simulink model "w2_warplab_trigger_proc"  (Simulink 7.7)
settings: Solver=ode45  StartTime=0.0  StopTime=1000  RelTol=1e-3
InitFcn:
  | w2_warplab_trigger_proc_init
StartFcn:
  | w2_warplab_trigger_proc_init
undefined symbols (not defined in the file or in its folder): gcbh, xlBlockLoadCallback, xlGetNormalizedPeriod
libraries: xbsIndex_r4 x819, simulink x1
(part 5 of 6)

== system w2_warplab_trigger_proc/Registers/Output Configuration Slice9 ==
  32b : Inport
  b0 : xbsIndex_r4/Slice  nbits=1  boolean_output=off  mode=Lower Bit Location + Width  bit1=0  base1=MSB of Input  bit0=0  base0=LSB of Input  dbl_ovrd=off  block_type=slice
  b1 : xbsIndex_r4/Slice  nbits=1  boolean_output=off  mode=Lower Bit Location + Width  bit1=0  base1=MSB of Input  bit0=1  base0=LSB of Input  dbl_ovrd=off  block_type=slice
  b16 : xbsIndex_r4/Slice  nbits=1  boolean_output=off  mode=Lower Bit Location + Width  bit1=0  base1=MSB of Input  bit0=16  base0=LSB of Input  dbl_ovrd=off  block_type=slice
  b17 : xbsIndex_r4/Slice  nbits=1  boolean_output=off  mode=Lower Bit Location + Width  bit1=0  base1=MSB of Input  bit0=17  base0=LSB of Input  dbl_ovrd=off  block_type=slice
  b18 : xbsIndex_r4/Slice  nbits=1  boolean_output=off  mode=Lower Bit Location + Width  bit1=0  base1=MSB of Input  bit0=18  base0=LSB of Input  dbl_ovrd=off  block_type=slice
  b19 : xbsIndex_r4/Slice  nbits=1  boolean_output=off  mode=Lower Bit Location + Width  bit1=0  base1=MSB of Input  bit0=19  base0=LSB of Input  dbl_ovrd=off  block_type=slice
  b2 : xbsIndex_r4/Slice  nbits=1  boolean_output=off  mode=Lower Bit Location + Width  bit1=0  base1=MSB of Input  bit0=2  base0=LSB of Input  dbl_ovrd=off  block_type=slice
  b20 : xbsIndex_r4/Slice  nbits=1  boolean_output=off  mode=Lower Bit Location + Width  bit1=0  base1=MSB of Input  bit0=20  base0=LSB of Input  dbl_ovrd=off  block_type=slice
  b21 : xbsIndex_r4/Slice  nbits=1  boolean_output=off  mode=Lower Bit Location + Width  bit1=0  base1=MSB of Input  bit0=21  base0=LSB of Input  dbl_ovrd=off  block_type=slice
  b22 : xbsIndex_r4/Slice  nbits=1  boolean_output=off  mode=Lower Bit Location + Width  bit1=0  base1=MSB of Input  bit0=22  base0=LSB of Input  dbl_ovrd=off  block_type=slice
  b23 : xbsIndex_r4/Slice  nbits=1  boolean_output=off  mode=Lower Bit Location + Width  bit1=0  base1=MSB of Input  bit0=23  base0=LSB of Input  dbl_ovrd=off  block_type=slice
  b24 : xbsIndex_r4/Slice  nbits=1  boolean_output=off  mode=Lower Bit Location + Width  bit1=0  base1=MSB of Input  bit0=24  base0=LSB of Input  dbl_ovrd=off  block_type=slice
  b3 : xbsIndex_r4/Slice  nbits=1  boolean_output=off  mode=Lower Bit Location + Width  bit1=0  base1=MSB of Input  bit0=3  base0=LSB of Input  dbl_ovrd=off  block_type=slice
  b4 : xbsIndex_r4/Slice  nbits=1  boolean_output=off  mode=Lower Bit Location + Width  bit1=0  base1=MSB of Input  bit0=4  base0=LSB of Input  dbl_ovrd=off  block_type=slice
  b5 : xbsIndex_r4/Slice  nbits=1  boolean_output=off  mode=Lower Bit Location + Width  bit1=0  base1=MSB of Input  bit0=5  base0=LSB of Input  dbl_ovrd=off  block_type=slice
  b6 : xbsIndex_r4/Slice  nbits=1  boolean_output=off  mode=Lower Bit Location + Width  bit1=0  base1=MSB of Input  bit0=6  base0=LSB of Input  dbl_ovrd=off  block_type=slice
  b7 : xbsIndex_r4/Slice  nbits=1  boolean_output=off  mode=Lower Bit Location + Width  bit1=0  base1=MSB of Input  bit0=7  base0=LSB of Input  dbl_ovrd=off  block_type=slice
  b8 : xbsIndex_r4/Slice  nbits=1  boolean_output=off  mode=Lower Bit Location + Width  bit1=0  base1=MSB of Input  bit0=8  base0=LSB of Input  dbl_ovrd=off  block_type=slice
  bool{1..18} (18 alike) : xbsIndex_r4/Convert  gui_display_data_type=Boolean  arith_type=Boolean  n_bits=16  bin_pt=14  float_type=Single  exp_bits=8  fraction_bits=24  quantization=Truncate  overflow=Wrap  en=off  latency=0  dbl_ovrd=off  pipeline=off  block_type=convert
  AND 0 : Outport
  AND 1 : Outport  Port=2
  AND 2 : Outport  Port=3
  AND 3 : Outport  Port=4
  AND 4 : Outport  Port=5
  AND 5 : Outport  Port=6
  AND 6 : Outport  Port=7
  AND 7 : Outport  Port=8
  AND 8 : Outport  Port=9
  OR 0 : Outport  Port=10
  OR 1 : Outport  Port=11
  OR 2 : Outport  Port=12
  OR 3 : Outport  Port=13
  OR 4 : Outport  Port=14
  OR 5 : Outport  Port=15
  OR 6 : Outport  Port=16
  OR 7 : Outport  Port=17
  OR 8 : Outport  Port=18
  wires:
  32b/1 -> b0/1, b1/1, b2/1, b3/1, b4/1, b5/1, b6/1, b7/1, b16/1, b17/1, b18/1, b19/1, b20/1, b21/1, b22/1, b23/1, b24/1, b8/1
  b0/1 -> bool2/1
  b1/1 -> bool1/1
  b2/1 -> bool3/1
  b3/1 -> bool4/1
  b4/1 -> bool5/1
  b5/1 -> bool6/1
  b6/1 -> bool7/1
  b7/1 -> bool8/1
  b16/1 -> bool9/1
  b17/1 -> bool10/1
  b18/1 -> bool11/1
  b19/1 -> bool12/1
  b20/1 -> bool13/1
  b21/1 -> bool14/1
  b22/1 -> bool15/1
  b23/1 -> bool16/1
  bool2/1 -> AND 0/1
  bool1/1 -> AND 1/1
  bool3/1 -> AND 2/1
  bool4/1 -> AND 3/1
  bool5/1 -> AND 4/1
  bool6/1 -> AND 5/1
  bool7/1 -> AND 6/1
  bool8/1 -> AND 7/1
  bool9/1 -> OR 0/1
  bool10/1 -> OR 1/1
  bool11/1 -> OR 2/1
  bool12/1 -> OR 3/1
  bool13/1 -> OR 4/1
  bool14/1 -> OR 5/1
  bool15/1 -> OR 6/1
  bool16/1 -> OR 7/1
  b8/1 -> bool17/1
  bool17/1 -> AND 8/1
  b24/1 -> bool18/1
  bool18/1 -> OR 8/1

== system w2_warplab_trigger_proc/Trigger Output 0/S-R Latch ==
  S : Inport
  R : Inport  Port=2
  Constant1 : xbsIndex_r4/Constant  const=1  gui_display_data_type=Fixed-point  arith_type=Unsigned  n_bits=1  bin_pt=0  preci_type=Single  exp_width=8  frac_width=24  explicit_period=off  period=1  equ=P=C  opselect=C  inp2=PCIN>>17  opr=+  inp1=P  carry=CIN  dbl_ovrd=off  block_type=constant
      settings: block_version=VER_STRING_GOES_HERE
  Convert1 : xbsIndex_r4/Convert  gui_display_data_type=Boolean  arith_type=Boolean  n_bits=16  bin_pt=14  float_type=Single  exp_bits=8  fraction_bits=24  quantization=Truncate  overflow=Wrap  en=off  latency=0  dbl_ovrd=off  pipeline=off  block_type=convert
  Convert2 : xbsIndex_r4/Convert  gui_display_data_type=Boolean  arith_type=Boolean  n_bits=16  bin_pt=14  float_type=Single  exp_bits=8  fraction_bits=24  quantization=Truncate  overflow=Wrap  en=off  latency=0  dbl_ovrd=off  pipeline=off  block_type=convert
  Register2 : xbsIndex_r4/Register  init=0  rst=on  en=on  dbl_ovrd=off  block_type=register
      settings: xl_area=[1 1 0 0 0 0 0]  block_version=VER_STRING_GOES_HERE
  Q : Outport
  wires:
  S/1 -> Convert2/1
  Register2/1 -> Q/1
  R/1 -> Convert1/1
  Constant1/1 -> Register2/1
  Convert1/1 -> Register2/2
  Convert2/1 -> Register2/3

== system w2_warplab_trigger_proc/Trigger Output 1/S-R Latch ==
  S : Inport
  R : Inport  Port=2
  Constant1 : xbsIndex_r4/Constant  const=1  gui_display_data_type=Fixed-point  arith_type=Unsigned  n_bits=1  bin_pt=0  preci_type=Single  exp_width=8  frac_width=24  explicit_period=off  period=1  equ=P=C  opselect=C  inp2=PCIN>>17  opr=+  inp1=P  carry=CIN  dbl_ovrd=off  block_type=constant
      settings: block_version=VER_STRING_GOES_HERE
  Convert1 : xbsIndex_r4/Convert  gui_display_data_type=Boolean  arith_type=Boolean  n_bits=16  bin_pt=14  float_type=Single  exp_bits=8  fraction_bits=24  quantization=Truncate  overflow=Wrap  en=off  latency=0  dbl_ovrd=off  pipeline=off  block_type=convert
  Convert2 : xbsIndex_r4/Convert  gui_display_data_type=Boolean  arith_type=Boolean  n_bits=16  bin_pt=14  float_type=Single  exp_bits=8  fraction_bits=24  quantization=Truncate  overflow=Wrap  en=off  latency=0  dbl_ovrd=off  pipeline=off  block_type=convert
  Register2 : xbsIndex_r4/Register  init=0  rst=on  en=on  dbl_ovrd=off  block_type=register
      settings: xl_area=[1 1 0 0 0 0 0]  block_version=VER_STRING_GOES_HERE
  Q : Outport
  wires:
  S/1 -> Convert2/1
  Register2/1 -> Q/1
  R/1 -> Convert1/1
  Constant1/1 -> Register2/1
  Convert1/1 -> Register2/2
  Convert2/1 -> Register2/3

== system w2_warplab_trigger_proc/Trigger Output 2/S-R Latch ==
  S : Inport
  R : Inport  Port=2
  Constant1 : xbsIndex_r4/Constant  const=1  gui_display_data_type=Fixed-point  arith_type=Unsigned  n_bits=1  bin_pt=0  preci_type=Single  exp_width=8  frac_width=24  explicit_period=off  period=1  equ=P=C  opselect=C  inp2=PCIN>>17  opr=+  inp1=P  carry=CIN  dbl_ovrd=off  block_type=constant
      settings: block_version=VER_STRING_GOES_HERE
  Convert1 : xbsIndex_r4/Convert  gui_display_data_type=Boolean  arith_type=Boolean  n_bits=16  bin_pt=14  float_type=Single  exp_bits=8  fraction_bits=24  quantization=Truncate  overflow=Wrap  en=off  latency=0  dbl_ovrd=off  pipeline=off  block_type=convert
  Convert2 : xbsIndex_r4/Convert  gui_display_data_type=Boolean  arith_type=Boolean  n_bits=16  bin_pt=14  float_type=Single  exp_bits=8  fraction_bits=24  quantization=Truncate  overflow=Wrap  en=off  latency=0  dbl_ovrd=off  pipeline=off  block_type=convert
  Register2 : xbsIndex_r4/Register  init=0  rst=on  en=on  dbl_ovrd=off  block_type=register
      settings: xl_area=[1 1 0 0 0 0 0]  block_version=VER_STRING_GOES_HERE
  Q : Outport
  wires:
  S/1 -> Convert2/1
  Register2/1 -> Q/1
  R/1 -> Convert1/1
  Constant1/1 -> Register2/1
  Convert1/1 -> Register2/2
  Convert2/1 -> Register2/3

== system w2_warplab_trigger_proc/Trigger Output 3/S-R Latch ==
  S : Inport
  R : Inport  Port=2
  Constant1 : xbsIndex_r4/Constant  const=1  gui_display_data_type=Fixed-point  arith_type=Unsigned  n_bits=1  bin_pt=0  preci_type=Single  exp_width=8  frac_width=24  explicit_period=off  period=1  equ=P=C  opselect=C  inp2=PCIN>>17  opr=+  inp1=P  carry=CIN  dbl_ovrd=off  block_type=constant
      settings: block_version=VER_STRING_GOES_HERE
  Convert1 : xbsIndex_r4/Convert  gui_display_data_type=Boolean  arith_type=Boolean  n_bits=16  bin_pt=14  float_type=Single  exp_bits=8  fraction_bits=24  quantization=Truncate  overflow=Wrap  en=off  latency=0  dbl_ovrd=off  pipeline=off  block_type=convert
  Convert2 : xbsIndex_r4/Convert  gui_display_data_type=Boolean  arith_type=Boolean  n_bits=16  bin_pt=14  float_type=Single  exp_bits=8  fraction_bits=24  quantization=Truncate  overflow=Wrap  en=off  latency=0  dbl_ovrd=off  pipeline=off  block_type=convert
  Register2 : xbsIndex_r4/Register  init=0  rst=on  en=on  dbl_ovrd=off  block_type=register
      settings: xl_area=[1 1 0 0 0 0 0]  block_version=VER_STRING_GOES_HERE
  Q : Outport
  wires:
  S/1 -> Convert2/1
  Register2/1 -> Q/1
  R/1 -> Convert1/1
  Constant1/1 -> Register2/1
  Convert1/1 -> Register2/2
  Convert2/1 -> Register2/3

== system w2_warplab_trigger_proc/Trigger Output 4/S-R Latch ==
  S : Inport
  R : Inport  Port=2
  Constant1 : xbsIndex_r4/Constant  const=1  gui_display_data_type=Fixed-point  arith_type=Unsigned  n_bits=1  bin_pt=0  preci_type=Single  exp_width=8  frac_width=24  explicit_period=off  period=1  equ=P=C  opselect=C  inp2=PCIN>>17  opr=+  inp1=P  carry=CIN  dbl_ovrd=off  block_type=constant
      settings: block_version=VER_STRING_GOES_HERE
  Convert1 : xbsIndex_r4/Convert  gui_display_data_type=Boolean  arith_type=Boolean  n_bits=16  bin_pt=14  float_type=Single  exp_bits=8  fraction_bits=24  quantization=Truncate  overflow=Wrap  en=off  latency=0  dbl_ovrd=off  pipeline=off  block_type=convert
  Convert2 : xbsIndex_r4/Convert  gui_display_data_type=Boolean  arith_type=Boolean  n_bits=16  bin_pt=14  float_type=Single  exp_bits=8  fraction_bits=24  quantization=Truncate  overflow=Wrap  en=off  latency=0  dbl_ovrd=off  pipeline=off  block_type=convert
  Register2 : xbsIndex_r4/Register  init=0  rst=on  en=on  dbl_ovrd=off  block_type=register
      settings: xl_area=[1 1 0 0 0 0 0]  block_version=VER_STRING_GOES_HERE
  Q : Outport
  wires:
  S/1 -> Convert2/1
  Register2/1 -> Q/1
  R/1 -> Convert1/1
  Constant1/1 -> Register2/1
  Convert1/1 -> Register2/2
  Convert2/1 -> Register2/3

== system w2_warplab_trigger_proc/Trigger Output 5/S-R Latch ==
  S : Inport
  R : Inport  Port=2
  Constant1 : xbsIndex_r4/Constant  const=1  gui_display_data_type=Fixed-point  arith_type=Unsigned  n_bits=1  bin_pt=0  preci_type=Single  exp_width=8  frac_width=24  explicit_period=off  period=1  equ=P=C  opselect=C  inp2=PCIN>>17  opr=+  inp1=P  carry=CIN  dbl_ovrd=off  block_type=constant
      settings: block_version=VER_STRING_GOES_HERE
  Convert1 : xbsIndex_r4/Convert  gui_display_data_type=Boolean  arith_type=Boolean  n_bits=16  bin_pt=14  float_type=Single  exp_bits=8  fraction_bits=24  quantization=Truncate  overflow=Wrap  en=off  latency=0  dbl_ovrd=off  pipeline=off  block_type=convert
  Convert2 : xbsIndex_r4/Convert  gui_display_data_type=Boolean  arith_type=Boolean  n_bits=16  bin_pt=14  float_type=Single  exp_bits=8  fraction_bits=24  quantization=Truncate  overflow=Wrap  en=off  latency=0  dbl_ovrd=off  pipeline=off  block_type=convert
  Register2 : xbsIndex_r4/Register  init=0  rst=on  en=on  dbl_ovrd=off  block_type=register
      settings: xl_area=[1 1 0 0 0 0 0]  block_version=VER_STRING_GOES_HERE
  Q : Outport
  wires:
  S/1 -> Convert2/1
  Register2/1 -> Q/1
  R/1 -> Convert1/1
  Constant1/1 -> Register2/1
  Convert1/1 -> Register2/2
  Convert2/1 -> Register2/3

== system w2_warplab_trigger_proc/Trigger Sources/AGC ==
  Constant2 : Constant  Value=0
  agc_done_in : xbsIndex_r4/Gateway In  gui_display_data_type=Boolean  arith_type=Boolean  n_bits=16  bin_pt=14  preci_type=Single  exp_width=8  frac_width=24  quantization="Round  (unbiased: +/- Inf)"  overflow=Saturate  period=1  dbl_ovrd=off  timing_constraint=None  locs_specified=off  LOCs={}  UseAsADC=off  ADCChannel='1'  inherit_from_input=off  hdl_port=on  block_type=gatewayin
  Trigger : Outport
  wires:
  agc_done_in/1 -> Trigger/1
  Constant2/1 -> agc_done_in/1

== system w2_warplab_trigger_proc/Trigger Sources/Debug 0 ==
  Logical : xbsIndex_r4/Logical  logical_function=AND  inputs=4  en=off  latency=0  precision=Full  arith_type=Unsigned  n_bits=16  bin_pt=0  align_bp=on  dbl_ovrd=off  block_type=logical
  Mux : xbsIndex_r4/Mux  inputs=2  en=off  latency=0  precision=Full  arith_type=Unsigned  n_bits=16  bin_pt=14  quantization=Truncate  overflow=Wrap  dbl_ovrd=off  block_type=mux
  Register{,1..4} (5 alike) : xbsIndex_r4/Register  init=0  rst=off  en=off  dbl_ovrd=off  block_type=register
  Step : Step  Time=50  SampleTime=0
  debug_0_in : xbsIndex_r4/Gateway In  gui_display_data_type=Boolean  arith_type=Boolean  n_bits=16  bin_pt=14  preci_type=Single  exp_width=8  frac_width=24  quantization="Round  (unbiased: +/- Inf)"  overflow=Saturate  period=1  dbl_ovrd=off  timing_constraint=None  locs_specified=off  LOCs={}  UseAsADC=off  ADCChannel='1'  inherit_from_input=off  hdl_port=on  block_type=gatewayin
  Trigger : Outport
  wires:
  Mux/1 -> Trigger/1
  debug_0_in/1 -> Register/1
  Register1/1 -> Register2/1, Logical/1
  Register2/1 -> Logical/2, Register3/1
  Register3/1 -> Register4/1, Logical/3
  [Debug_0_Debounce] -> Mux/1
  Register4/1 -> Logical/4
  Logical/1 -> Mux/3
  Step/1 -> debug_0_in/1
  Register/1 -> Mux/2, Register1/1

== system w2_warplab_trigger_proc/Trigger Sources/Debug 1 ==
  Constant2 : Constant  Value=0
  Logical : xbsIndex_r4/Logical  logical_function=AND  inputs=4  en=off  latency=0  precision=Full  arith_type=Unsigned  n_bits=16  bin_pt=0  align_bp=on  dbl_ovrd=off  block_type=logical
  Mux : xbsIndex_r4/Mux  inputs=2  en=off  latency=0  precision=Full  arith_type=Unsigned  n_bits=16  bin_pt=14  quantization=Truncate  overflow=Wrap  dbl_ovrd=off  block_type=mux
  Register{,1..4} (5 alike) : xbsIndex_r4/Register  init=0  rst=off  en=off  dbl_ovrd=off  block_type=register
  debug_1_in : xbsIndex_r4/Gateway In  gui_display_data_type=Boolean  arith_type=Boolean  n_bits=16  bin_pt=14  preci_type=Single  exp_width=8  frac_width=24  quantization="Round  (unbiased: +/- Inf)"  overflow=Saturate  period=1  dbl_ovrd=off  timing_constraint=None  locs_specified=off  LOCs={}  UseAsADC=off  ADCChannel='1'  inherit_from_input=off  hdl_port=on  block_type=gatewayin
  Trigger : Outport
  wires:
  Logical/1 -> Mux/3
  Register4/1 -> Logical/4
  [Debug_1_Debounce] -> Mux/1
  Register3/1 -> Logical/3, Register4/1
  Register2/1 -> Logical/2, Register3/1
  Register1/1 -> Logical/1, Register2/1
  debug_1_in/1 -> Register/1
  Mux/1 -> Trigger/1
  Register/1 -> Register1/1, Mux/2
  Constant2/1 -> debug_1_in/1

== system w2_warplab_trigger_proc/Trigger Sources/Debug 2 ==
  Constant2 : Constant  Value=0
  Logical : xbsIndex_r4/Logical  logical_function=AND  inputs=4  en=off  latency=0  precision=Full  arith_type=Unsigned  n_bits=16  bin_pt=0  align_bp=on  dbl_ovrd=off  block_type=logical
  Mux : xbsIndex_r4/Mux  inputs=2  en=off  latency=0  precision=Full  arith_type=Unsigned  n_bits=16  bin_pt=14  quantization=Truncate  overflow=Wrap  dbl_ovrd=off  block_type=mux
  Register{,1..4} (5 alike) : xbsIndex_r4/Register  init=0  rst=off  en=off  dbl_ovrd=off  block_type=register
  debug_2_in : xbsIndex_r4/Gateway In  gui_display_data_type=Boolean  arith_type=Boolean  n_bits=16  bin_pt=14  preci_type=Single  exp_width=8  frac_width=24  quantization="Round  (unbiased: +/- Inf)"  overflow=Saturate  period=1  dbl_ovrd=off  timing_constraint=None  locs_specified=off  LOCs={}  UseAsADC=off  ADCChannel='1'  inherit_from_input=off  hdl_port=on  block_type=gatewayin
  Trigger : Outport
  wires:
  Mux/1 -> Trigger/1
  debug_2_in/1 -> Register/1
  Register1/1 -> Register2/1, Logical/1
  Register2/1 -> Register3/1, Logical/2
  Register3/1 -> Register4/1, Logical/3
  [Debug_2_Debounce] -> Mux/1
  Register4/1 -> Logical/4
  Logical/1 -> Mux/3
  Register/1 -> Mux/2, Register1/1
  Constant2/1 -> debug_2_in/1

== system w2_warplab_trigger_proc/Trigger Sources/Debug 3 ==
  Constant2 : Constant  Value=0
  Logical : xbsIndex_r4/Logical  logical_function=AND  inputs=4  en=off  latency=0  precision=Full  arith_type=Unsigned  n_bits=16  bin_pt=0  align_bp=on  dbl_ovrd=off  block_type=logical
  Mux : xbsIndex_r4/Mux  inputs=2  en=off  latency=0  precision=Full  arith_type=Unsigned  n_bits=16  bin_pt=14  quantization=Truncate  overflow=Wrap  dbl_ovrd=off  block_type=mux
  Register{,1..4} (5 alike) : xbsIndex_r4/Register  init=0  rst=off  en=off  dbl_ovrd=off  block_type=register
  debug_3_in : xbsIndex_r4/Gateway In  gui_display_data_type=Boolean  arith_type=Boolean  n_bits=16  bin_pt=14  preci_type=Single  exp_width=8  frac_width=24  quantization="Round  (unbiased: +/- Inf)"  overflow=Saturate  period=1  dbl_ovrd=off  timing_constraint=None  locs_specified=off  LOCs={}  UseAsADC=off  ADCChannel='1'  inherit_from_input=off  hdl_port=on  block_type=gatewayin
  Trigger : Outport
  wires:
  Logical/1 -> Mux/3
  Register4/1 -> Logical/4
  [Debug_3_Debounce] -> Mux/1
  Register3/1 -> Logical/3, Register4/1
  Register2/1 -> Logical/2, Register3/1
  Register1/1 -> Logical/1, Register2/1
  debug_3_in/1 -> Register/1
  Mux/1 -> Trigger/1
  Register/1 -> Register1/1, Mux/2
  Constant2/1 -> debug_3_in/1

== system w2_warplab_trigger_proc/Trigger Sources/Energy ==
  16LSB : xbsIndex_r4/Slice  nbits=16  boolean_output=off  mode=Lower Bit Location + Width  bit1=0  base1=MSB of Input  bit0=0  base0=LSB of Input  dbl_ovrd=off  block_type=slice
  16MSB : xbsIndex_r4/Slice  nbits=16  boolean_output=off  mode=Lower Bit Location + Width  bit1=0  base1=MSB of Input  bit0=16  base0=LSB of Input  dbl_ovrd=off  block_type=slice
  AntA Detector : Subsystem
  AntB Detector : Subsystem
  AntC Detector : Subsystem
  AntD Detector : Subsystem
  Convert : xbsIndex_r4/Convert  gui_display_data_type=Boolean  arith_type=Boolean  n_bits=16  bin_pt=14  float_type=Single  exp_bits=8  fraction_bits=24  quantization=Truncate  overflow=Wrap  en=off  latency=0  dbl_ovrd=off  pipeline=off  block_type=convert
  Display : Display
      settings: Format=hex (Stored Integer)
  Display1 : Display
      settings: Format=hex (Stored Integer)
  Display2 : Display
      settings: Format=hex (Stored Integer)
  Gateway Out1 : xbsIndex_r4/Gateway Out  inherit_from_input=off  hdl_port=off  timing_constraint=None  locs_specified=off  LOCs={}  UseAsDAC=off  DACChannel='1'  block_type=gatewayout
  Gateway Out2 : xbsIndex_r4/Gateway Out  inherit_from_input=off  hdl_port=off  timing_constraint=None  locs_specified=off  LOCs={}  UseAsDAC=off  DACChannel='1'  block_type=gatewayout
  Gateway Out6 : xbsIndex_r4/Gateway Out  inherit_from_input=off  hdl_port=off  timing_constraint=None  locs_specified=off  LOCs={}  UseAsDAC=off  DACChannel='1'  block_type=gatewayout
  MIMO Logic : Subsystem
  Posedge : Subsystem
  Pulse Generator : DiscretePulseGenerator  PulseType=Time based  Period=16  PulseWidth=50
  RFA_RSSI : xbsIndex_r4/Gateway In  gui_display_data_type=Fixed-point  arith_type=Unsigned  n_bits=10  bin_pt=0  preci_type=Single  exp_width=8  frac_width=24  quantization=Truncate  overflow=Wrap  period=1  dbl_ovrd=off  timing_constraint=None  locs_specified=off  LOCs={}  UseAsADC=off  ADCChannel='1'  inherit_from_input=off  hdl_port=on  block_type=gatewayin
      settings: block_version=VER_STRING_GOES_HERE
  RFB_RSSI : xbsIndex_r4/Gateway In  gui_display_data_type=Fixed-point  arith_type=Unsigned  n_bits=10  bin_pt=0  preci_type=Single  exp_width=8  frac_width=24  quantization=Truncate  overflow=Wrap  period=1  dbl_ovrd=off  timing_constraint=None  locs_specified=off  LOCs={}  UseAsADC=off  ADCChannel='1'  inherit_from_input=off  hdl_port=on  block_type=gatewayin
      settings: infoedit="Gateway in block.  Converts inputs of type Simulink integer, double and fixed point to  Xilinx fixed point type.<P><P>Hardware notes:  In hardware these blocks become top level input ports."  block_version=VER_STRING_GOES_HERE
  RFC_RSSI : xbsIndex_r4/Gateway In  gui_display_data_type=Fixed-point  arith_type=Unsigned  n_bits=10  bin_pt=0  preci_type=Single  exp_width=8  frac_width=24  quantization=Truncate  overflow=Wrap  period=1  dbl_ovrd=off  timing_constraint=None  locs_specified=off  LOCs={}  UseAsADC=off  ADCChannel='1'  inherit_from_input=off  hdl_port=on  block_type=gatewayin
      settings: infoedit="Gateway in block.  Converts inputs of type Simulink integer, double and fixed point to  Xilinx fixed point type.<P><P>Hardware notes:  In hardware these blocks become top level input ports."  block_version=VER_STRING_GOES_HERE
  RFD_RSSI : xbsIndex_r4/Gateway In  gui_display_data_type=Fixed-point  arith_type=Unsigned  n_bits=10  bin_pt=0  preci_type=Single  exp_width=8  frac_width=24  quantization=Truncate  overflow=Wrap  period=1  dbl_ovrd=off  timing_constraint=None  locs_specified=off  LOCs={}  UseAsADC=off  ADCChannel='1'  inherit_from_input=off  hdl_port=on  block_type=gatewayin
      settings: infoedit="Gateway in block.  Converts inputs of type Simulink integer, double and fixed point to  Xilinx fixed point type.<P><P>Hardware notes:  In hardware these blocks become top level input ports."  block_version=VER_STRING_GOES_HERE
  RSSI_CLK : xbsIndex_r4/Gateway In  gui_display_data_type=Boolean  arith_type=Boolean  n_bits=10  bin_pt=0  preci_type=Single  exp_width=8  frac_width=24  quantization=Truncate  overflow=Wrap  period=1  dbl_ovrd=off  timing_constraint=None  locs_specified=off  LOCs={}  UseAsADC=off  ADCChannel='1'  inherit_from_input=off  hdl_port=on  block_type=gatewayin
      settings: block_version=VER_STRING_GOES_HERE
  Repeating Sequence : simulink/Sources/Repeating Sequence  SystemSampleTime=-1  rep_seq_t=[0 200 600]  rep_seq_y=[0 1023 0]
  b0 : xbsIndex_r4/Slice  nbits=1  boolean_output=off  mode=Lower Bit Location + Width  bit1=0  base1=MSB of Input  bit0=0  base0=LSB of Input  dbl_ovrd=off  block_type=slice
  b1 : xbsIndex_r4/Slice  nbits=1  boolean_output=off  mode=Lower Bit Location + Width  bit1=0  base1=MSB of Input  bit0=1  base0=LSB of Input  dbl_ovrd=off  block_type=slice
  b2 : xbsIndex_r4/Slice  nbits=1  boolean_output=off  mode=Lower Bit Location + Width  bit1=0  base1=MSB of Input  bit0=2  base0=LSB of Input  dbl_ovrd=off  block_type=slice
  b3 : xbsIndex_r4/Slice  nbits=1  boolean_output=off  mode=Lower Bit Location + Width  bit1=0  base1=MSB of Input  bit0=3  base0=LSB of Input  dbl_ovrd=off  block_type=slice
  b31 : xbsIndex_r4/Slice  nbits=1  boolean_output=off  mode=Lower Bit Location + Width  bit1=0  base1=MSB of Input  bit0=31  base0=LSB of Input  dbl_ovrd=off  block_type=slice
  b[15:8] : xbsIndex_r4/Slice  nbits=8  boolean_output=off  mode=Lower Bit Location + Width  bit1=0  base1=MSB of Input  bit0=8  base0=LSB of Input  dbl_ovrd=off  block_type=slice
  b[20:16] : xbsIndex_r4/Slice  nbits=5  boolean_output=off  mode=Lower Bit Location + Width  bit1=0  base1=MSB of Input  bit0=16  base0=LSB of Input  dbl_ovrd=off  block_type=slice
  b[7:0] : xbsIndex_r4/Slice  nbits=8  boolean_output=off  mode=Lower Bit Location + Width  bit1=0  base1=MSB of Input  bit0=0  base0=LSB of Input  dbl_ovrd=off  block_type=slice
  Trigger : Outport
  tag scope: pktDetMask_A=global, pktDetMask_B=global, pktDetMask_C=global, pktDetMask_D=global, pktDetReset=global, pktDet_duration_busy=global, pktDet_duration_idle=global, pktDet_energyThresh_busy=global, pktDet_energyThresh_idle=global, regPktDet_RSSIavgLength=global
  wires:
  AntA Detector/1(pktdet) -> MIMO Logic/1(Det A)
  [pktDetReset] -> Convert/1
  RFA_RSSI/1 -> AntA Detector/1(RSSI)
  [reg_pkt_det_config] -> b0/1, b1/1, b2/1, b3/1, Gateway Out6/1, b31/1
  [reg_pkt_det_thresh] -> 16LSB/1, 16MSB/1, Gateway Out1/1
  [reg_pkt_det_duration] -> b[7:0]/1, b[15:8]/1, b[20:16]/1, Gateway Out2/1
  16LSB/1 -> [pktDet_energyThresh_idle]
  16MSB/1 -> [pktDet_energyThresh_busy]
  b[7:0]/1 -> [pktDet_duration_idle]
  b[15:8]/1 -> [pktDet_duration_busy]
  b[20:16]/1 -> [regPktDet_RSSIavgLength]
  AntB Detector/1(pktdet) -> MIMO Logic/2(Det B)
  AntC Detector/1(pktdet) -> MIMO Logic/3(Det C)
  AntD Detector/1(pktdet) -> MIMO Logic/4(Det D)
  RFB_RSSI/1 -> AntB Detector/1(RSSI)
  RFC_RSSI/1 -> AntC Detector/1(RSSI)
  RFD_RSSI/1 -> AntD Detector/1(RSSI)
  Convert/1 -> AntA Detector/2(Reset), AntB Detector/2(Reset), AntC Detector/2(Reset), AntD Detector/2(Reset)
  MIMO Logic/1(PktDet) -> Trigger/1
  RSSI_CLK/1 -> Posedge/1(D)
  Posedge/1(Q) -> AntC Detector/3(En), AntD Detector/3(En), AntB Detector/3(En), AntA Detector/3(En)
  Repeating Sequence/1 -> RFA_RSSI/1, RFB_RSSI/1, RFC_RSSI/1, RFD_RSSI/1
  Pulse Generator/1 -> RSSI_CLK/1
  Gateway Out6/1 -> Display/1
  Gateway Out1/1 -> Display1/1
  Gateway Out2/1 -> Display2/1
  b0/1 -> [pktDetMask_A]
  b1/1 -> [pktDetMask_B]
  b2/1 -> [pktDetMask_C]
  b3/1 -> [pktDetMask_D]
  b31/1 -> [pktDetReset]

== system w2_warplab_trigger_proc/Trigger Sources/Eth A ==
  Trigger : Outport
  wires:
  [Eth_A_SW_Trig] -> Trigger/1

== system w2_warplab_trigger_proc/Trigger Sources/Software ==
  Trigger : Outport
  wires:
  [Software_Trig] -> Trigger/1

== system w2_warplab_trigger_proc/Trigger Sources/Energy/AntA Detector ==
  RSSI : Inport
  Reset : Inport  Port=2
  En : Inport  Port=3
  ASR : xbsIndex_r4/Addressable Shift Register  infer_latency=on  depth=2  initVector=[0]  en=on  dbl_ovrd=off  use_behavioral_HDL=off  Optimization=Resource  use_rpm=off  block_type=addrsr
      settings: infoedit="Delay of configurable length.  Any element in the delay line can be addressed and driven onto the output port.<br><br>Hardware notes: This block is implemented using SRL16s. If Virtex-4 or Spartan-3 device is used, multiple SRLC16s are cascaded together."  block_version=VER_STRING_GOES_HERE
  Busy Detection : Subsystem
  Delay : xbsIndex_r4/Delay  rst=off  infoeditControl=Selection of Reset will increase slice count due to use of real FFs and instead of SRLs  en=off  latency=2  dbl_ovrd=off  reg_retiming=off  block_type=delay
  Display : Display
  Gateway Out{,1..6} (7 alike) : xbsIndex_r4/Gateway Out  inherit_from_input=off  hdl_port=off  timing_constraint=None  locs_specified=off  LOCs={}  UseAsDAC=off  DACChannel='1'  block_type=gatewayout
      Gateway Out settings: infoedit="Gateway out block.  Converts Xilinx fixed point inputs into ouputs of type Simulink integer, double, or fixed point.<P><P>Hardware notes:  In hardware these blocks become top level output ports or are discarded, depending on how they are configured."  block_version=8.2
      Gateway Out1 settings: infoedit="Gateway out block.  Converts Xilinx fixed point inputs into ouputs of type Simulink integer, double, or fixed point.<P><P>Hardware notes:  In hardware these blocks become top level output ports or are discarded, depending on how they are configured."  block_version=8.2
      Gateway Out2 settings: infoedit="Gateway out block.  Converts Xilinx fixed point inputs into ouputs of type Simulink integer, double, or fixed point.<P><P>Hardware notes:  In hardware these blocks become top level output ports or are discarded, depending on how they are configured."  block_version=8.2
      Gateway Out3 settings: infoedit="Gateway out block.  Converts Xilinx fixed point inputs into ouputs of type Simulink integer, double, or fixed point.<P><P>Hardware notes:  In hardware these blocks become top level output ports or are discarded, depending on how they are configured."  block_version=8.2
      Gateway Out4 settings: infoedit="Gateway out block.  Converts Xilinx fixed point inputs into ouputs of type Simulink integer, double, or fixed point.<P><P>Hardware notes:  In hardware these blocks become top level output ports or are discarded, depending on how they are configured."  block_version=8.2
      Gateway Out5 settings: infoedit="Gateway out block.  Converts Xilinx fixed point inputs into ouputs of type Simulink integer, double, or fixed point.<P><P>Hardware notes:  In hardware these blocks become top level output ports or are discarded, depending on how they are configured."  block_version=8.2
  Idle Detection : Subsystem
  Logical : xbsIndex_r4/Logical  logical_function=AND  inputs=2  en=off  latency=0  precision=Full  arith_type=Unsigned  n_bits=16  bin_pt=0  align_bp=on  dbl_ovrd=off  block_type=logical
  Pkt Det Decision : Scope  NumInputPorts=6
      settings: TimeRange=1000  YMin=0~0~0~0~0~0  YMax=1000~15000~1~1~1~1
  Running Sum : Subsystem
  pktdet : Outport
  wires:
  Reset/1 -> Running Sum/2(reset), Idle Detection/2(Reset), Busy Detection/2(Reset)
  [regPktDet_RSSIavgLength] -> Running Sum/3(avglen), Gateway Out6/1
  Gateway Out/1 -> Pkt Det Decision/1  "RAWRSSI"
  Gateway Out1/1 -> Pkt Det Decision/2  "AVGRSSI"
  Gateway Out2/1 -> Pkt Det Decision/3  "IDLE"
  RSSI/1 -> Running Sum/1(RSSI), Gateway Out/1
  Running Sum/1(avg) -> Idle Detection/1(Avg RSSI), Busy Detection/1(Avg RSSI), Gateway Out1/1
  Idle Detection/1(Idle) -> Gateway Out2/1, Delay/1
  [pktDet_duration_busy] -> ASR/2
  ASR/1 -> Logical/1, Gateway Out5/1
  Busy Detection/1(Busy) -> Logical/2, Gateway Out3/1
  Logical/1 -> pktdet/1, Gateway Out4/1
  Gateway Out3/1 -> Pkt Det Decision/5  "BUSY"
  Gateway Out4/1 -> Pkt Det Decision/6  "DET"
  Gateway Out5/1 -> Pkt Det Decision/4  "IDLE DLY"
  Delay/1 -> ASR/1
  En/1 -> Running Sum/4(en), ASR/3, Idle Detection/3(en), Busy Detection/3(en)
  Gateway Out6/1 -> Display/1

== system w2_warplab_trigger_proc/Trigger Sources/Energy/AntB Detector ==
  RSSI : Inport
  Reset : Inport  Port=2
  En : Inport  Port=3
  ASR : xbsIndex_r4/Addressable Shift Register  infer_latency=on  depth=2  initVector=[0]  en=on  dbl_ovrd=off  use_behavioral_HDL=off  Optimization=Resource  use_rpm=off  block_type=addrsr
      settings: infoedit="Delay of configurable length.  Any element in the delay line can be addressed and driven onto the output port.<br><br>Hardware notes: This block is implemented using SRL16s. If Virtex-4 or Spartan-3 device is used, multiple SRLC16s are cascaded together."  block_version=VER_STRING_GOES_HERE
  Busy Detection : Subsystem
  Delay : xbsIndex_r4/Delay  rst=off  infoeditControl=Selection of Reset will increase slice count due to use of real FFs and instead of SRLs  en=off  latency=2  dbl_ovrd=off  reg_retiming=off  block_type=delay
  Gateway Out{,1..5} (6 alike) : xbsIndex_r4/Gateway Out  inherit_from_input=off  hdl_port=off  timing_constraint=None  locs_specified=off  LOCs={}  UseAsDAC=off  DACChannel='1'  block_type=gatewayout
      settings: infoedit="Gateway out block.  Converts Xilinx fixed point inputs into ouputs of type Simulink integer, double, or fixed point.<P><P>Hardware notes:  In hardware these blocks become top level output ports or are discarded, depending on how they are configured."  block_version=8.2
  Idle Detection : Subsystem
  Logical : xbsIndex_r4/Logical  logical_function=AND  inputs=2  en=off  latency=0  precision=Full  arith_type=Unsigned  n_bits=16  bin_pt=0  align_bp=on  dbl_ovrd=off  block_type=logical
  Pkt Det Decision : Scope  NumInputPorts=6
      settings: TimeRange=1000  YMin=0~0~0~0~0~0  YMax=1000~15000~1~1~1~1
  Running Sum : Subsystem
  pktdet : Outport
  wires:
  En/1 -> ASR/3, Idle Detection/3(en), Busy Detection/3(en), Running Sum/4(en)
  Delay/1 -> ASR/1
  Gateway Out5/1 -> Pkt Det Decision/4  "IDLE DLY"
  Gateway Out4/1 -> Pkt Det Decision/6  "DET"
  Gateway Out3/1 -> Pkt Det Decision/5  "BUSY"
  Logical/1 -> Gateway Out4/1, pktdet/1
  Busy Detection/1(Busy) -> Gateway Out3/1, Logical/2
  ASR/1 -> Gateway Out5/1, Logical/1
  [pktDet_duration_busy] -> ASR/2
  Idle Detection/1(Idle) -> Delay/1, Gateway Out2/1
  Running Sum/1(avg) -> Gateway Out1/1, Idle Detection/1(Avg RSSI), Busy Detection/1(Avg RSSI)
  RSSI/1 -> Gateway Out/1, Running Sum/1(RSSI)
  Gateway Out2/1 -> Pkt Det Decision/3  "IDLE"
  Gateway Out1/1 -> Pkt Det Decision/2  "AVGRSSI"
  Gateway Out/1 -> Pkt Det Decision/1  "RAWRSSI"
  [regPktDet_RSSIavgLength] -> Running Sum/3(avglen)
  Reset/1 -> Idle Detection/2(Reset), Busy Detection/2(Reset), Running Sum/2(reset)

== system w2_warplab_trigger_proc/Trigger Sources/Energy/AntC Detector ==
  RSSI : Inport
  Reset : Inport  Port=2
  En : Inport  Port=3
  ASR : xbsIndex_r4/Addressable Shift Register  infer_latency=on  depth=2  initVector=[0]  en=on  dbl_ovrd=off  use_behavioral_HDL=off  Optimization=Resource  use_rpm=off  block_type=addrsr
      settings: infoedit="Delay of configurable length.  Any element in the delay line can be addressed and driven onto the output port.<br><br>Hardware notes: This block is implemented using SRL16s. If Virtex-4 or Spartan-3 device is used, multiple SRLC16s are cascaded together."  block_version=VER_STRING_GOES_HERE
  Busy Detection : Subsystem
  Delay : xbsIndex_r4/Delay  rst=off  infoeditControl=Selection of Reset will increase slice count due to use of real FFs and instead of SRLs  en=off  latency=2  dbl_ovrd=off  reg_retiming=off  block_type=delay
  Gateway Out{,1..5} (6 alike) : xbsIndex_r4/Gateway Out  inherit_from_input=off  hdl_port=off  timing_constraint=None  locs_specified=off  LOCs={}  UseAsDAC=off  DACChannel='1'  block_type=gatewayout
      settings: infoedit="Gateway out block.  Converts Xilinx fixed point inputs into ouputs of type Simulink integer, double, or fixed point.<P><P>Hardware notes:  In hardware these blocks become top level output ports or are discarded, depending on how they are configured."  block_version=8.2
  Idle Detection : Subsystem
  Logical : xbsIndex_r4/Logical  logical_function=AND  inputs=2  en=off  latency=0  precision=Full  arith_type=Unsigned  n_bits=16  bin_pt=0  align_bp=on  dbl_ovrd=off  block_type=logical
  Pkt Det Decision : Scope  NumInputPorts=6
      settings: TimeRange=1000  YMin=0~0~0~0~0~0  YMax=1000~15000~1~1~1~1
  Running Sum : Subsystem
  pktdet : Outport
  wires:
  Reset/1 -> Running Sum/2(reset), Busy Detection/2(Reset), Idle Detection/2(Reset)
  [regPktDet_RSSIavgLength] -> Running Sum/3(avglen)
  Gateway Out/1 -> Pkt Det Decision/1  "RAWRSSI"
  Gateway Out1/1 -> Pkt Det Decision/2  "AVGRSSI"
  Gateway Out2/1 -> Pkt Det Decision/3  "IDLE"
  RSSI/1 -> Running Sum/1(RSSI), Gateway Out/1
  Running Sum/1(avg) -> Busy Detection/1(Avg RSSI), Idle Detection/1(Avg RSSI), Gateway Out1/1
  Idle Detection/1(Idle) -> Gateway Out2/1, Delay/1
  [pktDet_duration_busy] -> ASR/2
  ASR/1 -> Logical/1, Gateway Out5/1
  Busy Detection/1(Busy) -> Logical/2, Gateway Out3/1
  Logical/1 -> pktdet/1, Gateway Out4/1
  Gateway Out3/1 -> Pkt Det Decision/5  "BUSY"
  Gateway Out4/1 -> Pkt Det Decision/6  "DET"
  Gateway Out5/1 -> Pkt Det Decision/4  "IDLE DLY"
  Delay/1 -> ASR/1
  En/1 -> Running Sum/4(en), ASR/3, Busy Detection/3(en), Idle Detection/3(en)

== system w2_warplab_trigger_proc/Trigger Sources/Energy/AntD Detector ==
  RSSI : Inport
  Reset : Inport  Port=2
  En : Inport  Port=3
  ASR : xbsIndex_r4/Addressable Shift Register  infer_latency=on  depth=2  initVector=[0]  en=on  dbl_ovrd=off  use_behavioral_HDL=off  Optimization=Resource  use_rpm=off  block_type=addrsr
      settings: infoedit="Delay of configurable length.  Any element in the delay line can be addressed and driven onto the output port.<br><br>Hardware notes: This block is implemented using SRL16s. If Virtex-4 or Spartan-3 device is used, multiple SRLC16s are cascaded together."  block_version=VER_STRING_GOES_HERE
  Busy Detection : Subsystem
  Delay : xbsIndex_r4/Delay  rst=off  infoeditControl=Selection of Reset will increase slice count due to use of real FFs and instead of SRLs  en=off  latency=2  dbl_ovrd=off  reg_retiming=off  block_type=delay
  Gateway Out{,1..5} (6 alike) : xbsIndex_r4/Gateway Out  inherit_from_input=off  hdl_port=off  timing_constraint=None  locs_specified=off  LOCs={}  UseAsDAC=off  DACChannel='1'  block_type=gatewayout
      settings: infoedit="Gateway out block.  Converts Xilinx fixed point inputs into ouputs of type Simulink integer, double, or fixed point.<P><P>Hardware notes:  In hardware these blocks become top level output ports or are discarded, depending on how they are configured."  block_version=8.2
  Idle Detection : Subsystem
  Logical : xbsIndex_r4/Logical  logical_function=AND  inputs=2  en=off  latency=0  precision=Full  arith_type=Unsigned  n_bits=16  bin_pt=0  align_bp=on  dbl_ovrd=off  block_type=logical
  Pkt Det Decision : Scope  NumInputPorts=6
      settings: TimeRange=1000  YMin=0~0~0~0~0~0  YMax=1000~15000~1~1~1~1
  Running Sum : Subsystem
  pktdet : Outport
  wires:
  En/1 -> ASR/3, Idle Detection/3(en), Busy Detection/3(en), Running Sum/4(en)
  Delay/1 -> ASR/1
  Gateway Out5/1 -> Pkt Det Decision/4  "IDLE DLY"
  Gateway Out4/1 -> Pkt Det Decision/6  "DET"
  Gateway Out3/1 -> Pkt Det Decision/5  "BUSY"
  Logical/1 -> Gateway Out4/1, pktdet/1
  Busy Detection/1(Busy) -> Gateway Out3/1, Logical/2
  ASR/1 -> Gateway Out5/1, Logical/1
  [pktDet_duration_busy] -> ASR/2
  Idle Detection/1(Idle) -> Delay/1, Gateway Out2/1
  Running Sum/1(avg) -> Gateway Out1/1, Idle Detection/1(Avg RSSI), Busy Detection/1(Avg RSSI)
  RSSI/1 -> Gateway Out/1, Running Sum/1(RSSI)
  Gateway Out2/1 -> Pkt Det Decision/3  "IDLE"
  Gateway Out1/1 -> Pkt Det Decision/2  "AVGRSSI"
  Gateway Out/1 -> Pkt Det Decision/1  "RAWRSSI"
  [regPktDet_RSSIavgLength] -> Running Sum/3(avglen)
  Reset/1 -> Idle Detection/2(Reset), Busy Detection/2(Reset), Running Sum/2(reset)

== system w2_warplab_trigger_proc/Trigger Sources/Energy/MIMO Logic ==
  Det A : Inport
  Det B : Inport  Port=2
  Det C : Inport  Port=3
  Det D : Inport  Port=4
  Convert{1..8} (8 alike) : xbsIndex_r4/Convert  gui_display_data_type=Fixed-point  arith_type=Unsigned  n_bits=1  bin_pt=0  float_type=Single  exp_bits=8  fraction_bits=24  quantization=Truncate  overflow=Flag as error  en=off  latency=0  dbl_ovrd=off  pipeline=off  block_type=convert
      settings: block_version=10.1.3
  Logical{,1,3..4} (4 alike) : xbsIndex_r4/Logical  logical_function=AND  inputs=2  en=off  latency=0  precision=Full  arith_type=Unsigned  n_bits=16  bin_pt=0  align_bp=on  dbl_ovrd=off  block_type=logical
  Logical2 : xbsIndex_r4/Logical  logical_function=OR  inputs=4  en=off  latency=0  precision=Full  arith_type=Unsigned  n_bits=16  bin_pt=0  align_bp=on  dbl_ovrd=off  block_type=logical
  PktDet : Outport
  wires:
  [pktDetMask_A] -> Convert2/1
  [pktDetMask_B] -> Convert3/1
  Det A/1 -> Convert7/1
  Det B/1 -> Convert1/1
  Convert7/1 -> Logical/1
  Convert2/1 -> Logical/2
  Convert1/1 -> Logical1/1
  Convert3/1 -> Logical1/2
  Logical/1 -> Logical2/1
  Logical1/1 -> Logical2/2
  Logical2/1 -> PktDet/1
  [pktDetMask_C] -> Convert5/1
  Det C/1 -> Convert4/1
  Convert4/1 -> Logical3/1
  Convert5/1 -> Logical3/2
  Logical3/1 -> Logical2/3
  [pktDetMask_D] -> Convert8/1
  Det D/1 -> Convert6/1
  Convert6/1 -> Logical4/1
  Convert8/1 -> Logical4/2
  Logical4/1 -> Logical2/4

== system w2_warplab_trigger_proc/Trigger Sources/Energy/Posedge ==
  D : Inport
  Delay : xbsIndex_r4/Delay  rst=off  infoeditControl=Selection of Reset will increase slice count due to use of real FFs and instead of SRLs  en=off  latency=1  dbl_ovrd=off  reg_retiming=off  block_type=delay
      settings: infoedit=Hardware notes: A delay line is a chain, each link of which is an SRL16 followed by a flip-flop. If register retiming is enabled, the delay line is a chain of flip-flops.  block_version=8.2
  Inverter : xbsIndex_r4/Inverter  en=off  latency=0  dbl_ovrd=off  block_type=inv
      settings: block_version=8.2
  Logical : xbsIndex_r4/Logical  logical_function=AND  inputs=2  en=off  latency=0  precision=Full  arith_type=Unsigned  n_bits=16  bin_pt=0  align_bp=on  dbl_ovrd=off  block_type=logical
      settings: block_version=8.2
  Q : Outport
  wires:
  D/1 -> Inverter/1, Logical/1
  Inverter/1 -> Delay/1
  Delay/1 -> Logical/2
  Logical/1 -> Q/1

== system w2_warplab_trigger_proc/Trigger Sources/Energy/AntA Detector/Busy Detection ==
  Avg RSSI : Inport
  Reset : Inport  Port=2
  en : Inport  Port=3
  Convert1 : xbsIndex_r4/Convert  gui_display_data_type=Fixed-point  arith_type=Unsigned  n_bits=1  bin_pt=0  float_type=Single  exp_bits=8  fraction_bits=24  quantization=Truncate  overflow=Wrap  en=off  latency=0  dbl_ovrd=off  pipeline=off  block_type=convert
      settings: block_version=VER_STRING_GOES_HERE
  Counter1 : xbsIndex_r4/Counter  cnt_type=Free Running  cnt_to=Inf  operation=Up  start_count=0  cnt_by_val=1  arith_type=Unsigned  n_bits=11  bin_pt=0  load_pin=off  rst=on  en=on  explicit_period=off  period=4  dbl_ovrd=off  use_behavioral_HDL=off  implementation=Fabric  use_rpm=off  block_type=counter
  Display : Display
  Display1 : Display
  Gateway Out1 : xbsIndex_r4/Gateway Out  inherit_from_input=off  hdl_port=off  timing_constraint=None  locs_specified=off  LOCs={}  UseAsDAC=off  DACChannel='1'  block_type=gatewayout
  Gateway Out6 : xbsIndex_r4/Gateway Out  inherit_from_input=off  hdl_port=off  timing_constraint=None  locs_specified=off  LOCs={}  UseAsDAC=off  DACChannel='1'  block_type=gatewayout
  Inverter1 : xbsIndex_r4/Inverter  en=off  latency=0  dbl_ovrd=off  block_type=inv
      settings: xl_area=[0 0 0 0 0 0 0]  block_version=8.2
  Logical : xbsIndex_r4/Logical  logical_function=AND  inputs=2  en=off  latency=0  precision=Full  arith_type=Unsigned  n_bits=16  bin_pt=0  align_bp=on  dbl_ovrd=off  block_type=logical
  Logical1 : xbsIndex_r4/Logical  logical_function=OR  inputs=2  en=off  latency=0  precision=Full  arith_type=Unsigned  n_bits=16  bin_pt=0  align_bp=on  dbl_ovrd=off  block_type=logical
  Relational2 : xbsIndex_r4/Relational  mode=a>b  en=off  latency=0  dbl_ovrd=off  block_type=relational
      settings: block_version=VER_STRING_GOES_HERE
  Relational3 : xbsIndex_r4/Relational  mode=a>b  en=off  latency=0  dbl_ovrd=off  block_type=relational
      settings: block_version=VER_STRING_GOES_HERE
  S-R Latch : Subsystem
  Busy : Outport
  wires:
  [pktDet_energyThresh_busy] -> Relational2/2, Gateway Out6/1
  Reset/1 -> Logical1/1
  Logical1/1 -> Counter1/1, S-R Latch/1(R)
  Inverter1/1 -> Logical1/2
  Counter1/1 -> Relational3/1
  [pktDet_duration_busy] -> Relational3/2, Gateway Out1/1
  Relational3/1 -> S-R Latch/2(S)
  S-R Latch/1(Q) -> Convert1/1
  Avg RSSI/1 -> Relational2/1
  Convert1/1 -> Busy/1
  Logical/1 -> Counter1/2
  Relational2/1 -> Logical/1, Inverter1/1
  en/1 -> Logical/2
  Gateway Out6/1 -> Display/1
  Gateway Out1/1 -> Display1/1

== system w2_warplab_trigger_proc/Trigger Sources/Energy/AntA Detector/Idle Detection ==
  Avg RSSI : Inport
  Reset : Inport  Port=2
  en : Inport  Port=3
  Convert1 : xbsIndex_r4/Convert  gui_display_data_type=Fixed-point  arith_type=Unsigned  n_bits=1  bin_pt=0  float_type=Single  exp_bits=8  fraction_bits=24  quantization=Truncate  overflow=Wrap  en=off  latency=0  dbl_ovrd=off  pipeline=off  block_type=convert
      settings: block_version=VER_STRING_GOES_HERE
  Counter1 : xbsIndex_r4/Counter  cnt_type=Free Running  cnt_to=Inf  operation=Up  start_count=0  cnt_by_val=1  arith_type=Unsigned  n_bits=11  bin_pt=0  load_pin=off  rst=on  en=on  explicit_period=off  period=4  dbl_ovrd=off  use_behavioral_HDL=off  implementation=Fabric  use_rpm=off  block_type=counter
  Display : Display
  Display1 : Display
  Gateway Out1 : xbsIndex_r4/Gateway Out  inherit_from_input=off  hdl_port=off  timing_constraint=None  locs_specified=off  LOCs={}  UseAsDAC=off  DACChannel='1'  block_type=gatewayout
  Gateway Out6 : xbsIndex_r4/Gateway Out  inherit_from_input=off  hdl_port=off  timing_constraint=None  locs_specified=off  LOCs={}  UseAsDAC=off  DACChannel='1'  block_type=gatewayout
  Inverter1 : xbsIndex_r4/Inverter  en=off  latency=0  dbl_ovrd=off  block_type=inv
      settings: xl_area=[0 0 0 0 0 0 0]  block_version=8.2
  Logical : xbsIndex_r4/Logical  logical_function=AND  inputs=2  en=off  latency=0  precision=Full  arith_type=Unsigned  n_bits=16  bin_pt=0  align_bp=on  dbl_ovrd=off  block_type=logical
  Logical1 : xbsIndex_r4/Logical  logical_function=OR  inputs=2  en=off  latency=0  precision=Full  arith_type=Unsigned  n_bits=16  bin_pt=0  align_bp=on  dbl_ovrd=off  block_type=logical
  Relational2 : xbsIndex_r4/Relational  mode=a<b  en=off  latency=0  dbl_ovrd=off  block_type=relational
      settings: block_version=VER_STRING_GOES_HERE
  Relational3 : xbsIndex_r4/Relational  mode=a>b  en=off  latency=0  dbl_ovrd=off  block_type=relational
      settings: block_version=VER_STRING_GOES_HERE
  S-R Latch : Subsystem
  Idle : Outport
  wires:
  Convert1/1 -> Idle/1
  Avg RSSI/1 -> Relational2/1
  S-R Latch/1(Q) -> Convert1/1
  Relational3/1 -> S-R Latch/2(S)
  [pktDet_duration_idle] -> Relational3/2, Gateway Out1/1
  Counter1/1 -> Relational3/1
  Inverter1/1 -> Logical1/2
  Logical1/1 -> Counter1/1, S-R Latch/1(R)
  Reset/1 -> Logical1/1
  Relational2/1 -> Logical/1, Inverter1/1
  [pktDet_energyThresh_idle] -> Relational2/2, Gateway Out6/1
  en/1 -> Logical/2
  Logical/1 -> Counter1/2
  Gateway Out6/1 -> Display/1
  Gateway Out1/1 -> Display1/1

== system w2_warplab_trigger_proc/Trigger Sources/Energy/AntA Detector/Running Sum ==
  note: This block impelemnts a variable-length running sum.
      | For a sum y(n) of the previous N samples of sequence x(n), it implements
      | y(n) = y(n-1) + x(n) - x(n-N)
      | This requires a careful reset procedure, where the full shift register
      | is zerored out. Otherwise the feedback-based sum stops working.
  RSSI : Inport
  reset : Inport  Port=2
  avglen : Inport  Port=3
  en : Inport  Port=4
  ASR : xbsIndex_r4/Addressable Shift Register  infer_latency=on  depth=2  initVector=[0]  en=on  dbl_ovrd=off  use_behavioral_HDL=off  Optimization=Resource  use_rpm=off  block_type=addrsr
      settings: infoedit="Delay of configurable length.  Any element in the delay line can be addressed and driven onto the output port.<br><br>Hardware notes: This block is implemented using SRL16s. If Virtex-4 or Spartan-3 device is used, multiple SRLC16s are cascaded together."  block_version=VER_STRING_GOES_HERE
  Accumulator : xbsIndex_r4/Accumulator  operation=Add  n_bits=17  overflow=Flag as error  scale=1  rst=on  infoeditControl=reset for floating point data type must be asserted for a minimum of 2 cycles  hasbypass=off  en=on  latency=0  dbl_ovrd=off  msb_inp=100  msb=100  lsb=-100  use_behavioral_HDL=on  implementation=Fabric  block_type=accum
      settings: block_version=VER_STRING_GOES_HERE
  AddSub : xbsIndex_r4/AddSub  mode=Subtraction  use_carryin=off  use_carryout=off  en=off  latency=0  precision=Full  arith_type=Unsigned  n_bits=10  bin_pt=0  quantization=Truncate  overflow=Wrap  dbl_ovrd=off  use_behavioral_HDL=off  hw_selection=Fabric  pipelined=off  use_rpm=on  block_type=addsub
      settings: block_version=VER_STRING_GOES_HERE
  Convert7 : xbsIndex_r4/Convert  gui_display_data_type=Fixed-point  arith_type=Unsigned  n_bits=17  bin_pt=0  float_type=Single  exp_bits=8  fraction_bits=24  quantization=Truncate  overflow=Saturate  en=off  latency=0  dbl_ovrd=off  pipeline=off  block_type=convert
      settings: block_version=10.1.3
  Logical : xbsIndex_r4/Logical  logical_function=OR  inputs=2  en=off  latency=0  precision=Full  arith_type=Unsigned  n_bits=16  bin_pt=0  align_bp=on  dbl_ovrd=off  block_type=logical
  Long Reset Gen : Subsystem
  Register : xbsIndex_r4/Register  init=0  rst=on  en=off  dbl_ovrd=off  block_type=register
      settings: block_version=VER_STRING_GOES_HERE
  avg : Outport
  wires:
  ASR/1 -> AddSub/2
  AddSub/1 -> Accumulator/1
  Register/1 -> ASR/1, AddSub/1
  avglen/1 -> ASR/2, Long Reset Gen/1(duration)
  RSSI/1 -> Register/1
  Accumulator/1 -> Convert7/1
  Logical/1 -> Register/2, Accumulator/2
  reset/1 -> Long Reset Gen/2(reset_in), Logical/2
  Long Reset Gen/1(reset_out) -> Logical/1
  Convert7/1 -> avg/1
  en/1 -> ASR/3, Accumulator/3
